simulink model "main_simulation_without_FKw"  (R2015a)
settings: Solver=ode45  StartTime=0.0  StopTime=10  FixedStep=1e-4  MaxStep=1e-3  RelTol=1e-3
values from neighbouring files (symbols this model uses):
  Ab11 = Ab(1:qw,1:qw)    [main_new.m]
  Ab12 = Ab(1:qw,qw+1:end)    [main_new.m]
  Ap = A    [main_new.m]
  Bb1 = Bb(1:qw,:)    [main_new.m]
  Bp = B    [main_new.m]
  Cb1p = (Cb1'*Cb1)^-1*Cb1'    [main_new.m]
  Cb2 = Cb(:,qw+1:end)    [main_new.m]
  Cp = C    [main_new.m]
  Ct = M*(eye(p)-Cb1*Cb1p)*Cb2    [main_new.m]
  Hp = H    [main_new.m]
  Ht = M*(eye(p)-Cb1*Cb1p)    [main_new.m]
  Kw = [0.158157916499 0.63846121775 -0.50742483629]    [Kw.mat]
  Kx = [0.978793467395 0.115253740456 -0.0372496439283 0.23631932633 2.68523757626 0.686096731216 0.555565644056 0.104452817235 0.744612452854 0.95412117755 0.434401201084 2.92090282506 ... (18 elements, 3x6)]    [Kx.mat]
  L = [732.974875612  -277.124666785; -145.685949536  40.2310279193; -21.3176025114  5.29309640103; -7.2125257354  1.1132328988; -36.4024893883  14.5426348186]    [L.mat]
  N = [-9.05549588116 -0.0761441556143 -0.0825387256676 0.135276633069 -0.0642378069483 -0.0761441556143 -9.64406895175 0.00880586634764 0.827985535249 0.695939837272 -0.0825387256676 0.00880586634764 ... (25 elements, 5x5)]    [N.mat]
  Q1 = Q(:,1:qw)    [main_new.m]
  Q2 = Q(:,qw+1:end)    [main_new.m]
  Sigma1 = Sigmaw(1:qw,:)    [main_new.m]
undefined symbols (not defined in the file or in its folder): C, J
libraries: dsparch4 x1
settings Model: Creator=p4wp4w  LastModifiedBy=p4wp4w

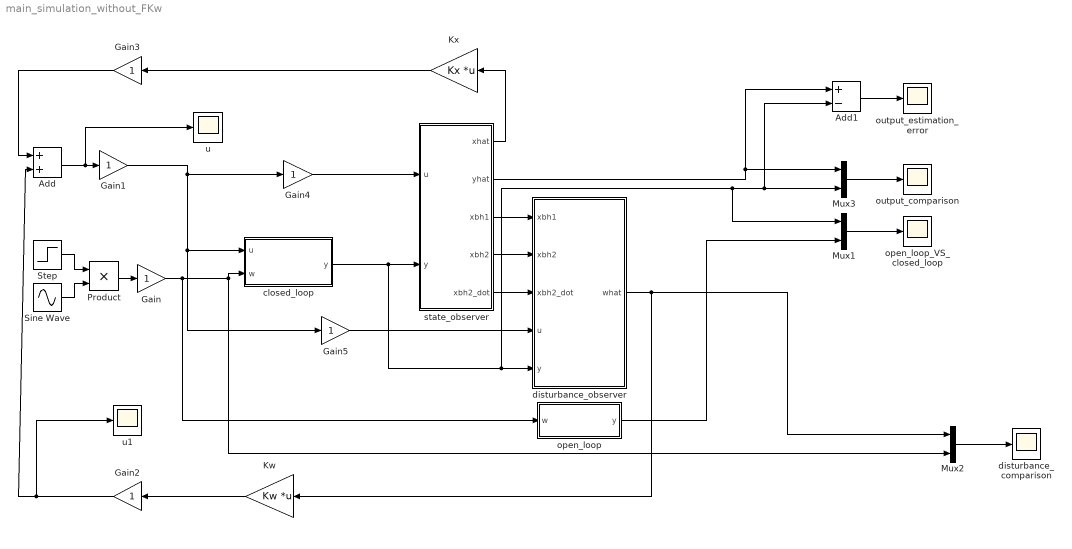
== system main_simulation_without_FKw ==
  Add : Sum
  Add1 : Sum  Inputs=+-
  Gain{,1..5} (6 alike) : Gain
  Kw : Gain  Gain=Kw  Multiplication=Matrix(K*u)
  Kx : Gain  Gain=Kx  Multiplication=Matrix(K*u)
  Mux1 : Mux  Inputs=2
  Mux2 : Mux  Inputs=2
  Mux3 : Mux  Inputs=2
  Product : Product
  Sine Wave : Sin  Frequency=10  SampleTime=0
  Step : Step  Time=5  Before=8  After=0  SampleTime=0
  closed_loop : Subsystem
  disturbance_comparison : Scope
      settings: YMin=-15  YMax=15
  disturbance_observer : Subsystem
  open_loop : Subsystem
  open_loop_VS_closed_loop : Scope
      settings: ShowLegends=on  YMin=-2.5e+09  YMax=3e+10  SaveName=ScopeData4
  output_comparison : Scope
      settings: YMin=-0.0024  YMax=-2.1684e-19
  output_estimation_error : Scope
      settings: YMin=-0.0024  YMax=-2.1684e-19  SaveName=ScopeData3
  state_observer : Subsystem
  u : Scope
      settings: SaveName=ScopeData2
  u1 : Scope
      settings: YMin=-2.5e+33  YMax=8.5e+33  SaveName=ScopeData5
  wires:
  Gain1/1 -> Gain5/1, closed_loop/1(u), Gain4/1
  closed_loop/1(y) -> Mux1/1, Add1/2, Mux3/2, disturbance_observer/5(y), state_observer/2(y)
  Mux2/1 -> disturbance_comparison/1
  state_observer/3(xbh1) -> disturbance_observer/1(xbh1)
  state_observer/4(xbh2) -> disturbance_observer/2(xbh2)
  state_observer/5(xbh2_dot) -> disturbance_observer/3(xbh2_dot)
  Mux3/1 -> output_comparison/1
  state_observer/2(yhat) -> Add1/1, Mux3/1
  disturbance_observer/1(what) -> Kw/1, Mux2/1
  Gain/1 -> open_loop/1(w), Mux2/2, closed_loop/2(w)
  state_observer/1(xhat) -> Kx/1
  Add/1 -> u/1, Gain1/1
  Kx/1 -> Gain3/1
  Kw/1 -> Gain2/1
  Gain2/1 -> u1/1, Add/2
  Gain3/1 -> Add/1
  Add1/1 -> output_estimation_error/1
  open_loop/1(y) -> Mux1/2
  Mux1/1 -> open_loop_VS_closed_loop/1
  Product/1 -> Gain/1
  Step/1 -> Product/1
  Sine Wave/1 -> Product/2
  Gain4/1 -> state_observer/1(u)
  Gain5/1 -> disturbance_observer/4(u)

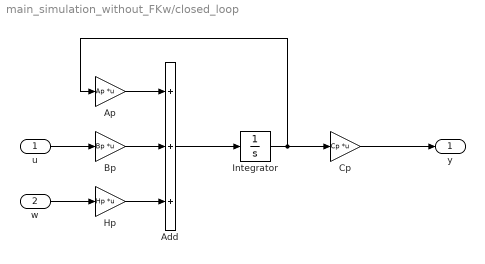
== system main_simulation_without_FKw/closed_loop ==
  u : Inport
  w : Inport  Port=2
  Add : Sum  Inputs=+++
  Ap : Gain  Gain=Ap  Multiplication=Matrix(K*u)
  Bp : Gain  Gain=Bp  Multiplication=Matrix(K*u)
  Cp : Gain  Gain=Cp  Multiplication=Matrix(K*u)
  Hp : Gain  Gain=Hp  Multiplication=Matrix(K*u)
  Integrator : Integrator
  y : Outport
  wires:
  w/1 -> Hp/1
  u/1 -> Bp/1
  Add/1 -> Integrator/1
  Bp/1 -> Add/2
  Integrator/1 -> Cp/1, Ap/1
  Ap/1 -> Add/1
  Hp/1 -> Add/3
  Cp/1 -> y/1

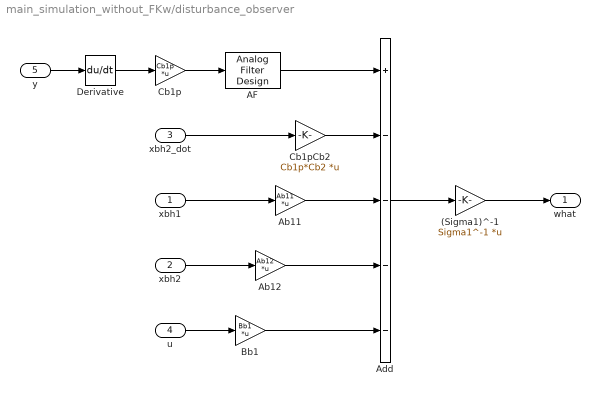
== system main_simulation_without_FKw/disturbance_observer ==
  xbh1 : Inport
  xbh2 : Inport  Port=2
  xbh2_dot : Inport  Port=3
  u : Inport  Port=4
  y : Inport  Port=5
  (Sigma1)^-1 : Gain  Gain=Sigma1^-1  Multiplication=Matrix(K*u)
  AF : dsparch4/Analog Filter Design  method=Butterworth  filttype=Lowpass  N=2  Wlo=30  Whi=80  Rp=2  Rs=40
  Ab11 : Gain  Gain=Ab11  Multiplication=Matrix(K*u)
  Ab12 : Gain  Gain=Ab12  Multiplication=Matrix(K*u)
  Add : Sum  Inputs=+----
  Bb1 : Gain  Gain=Bb1  Multiplication=Matrix(K*u)
  Cb1p : Gain  Gain=Cb1p  Multiplication=Matrix(K*u)
  Cb1pCb2 : Gain  Gain=Cb1p*Cb2  Multiplication=Matrix(K*u)
  Derivative : Derivative
  what : Outport
  wires:
  (Sigma1)^-1/1 -> what/1
  y/1 -> Derivative/1
  Derivative/1 -> Cb1p/1
  Add/1 -> (Sigma1)^-1/1
  Cb1pCb2/1 -> Add/2
  xbh2_dot/1 -> Cb1pCb2/1
  Ab11/1 -> Add/3
  xbh1/1 -> Ab11/1
  Ab12/1 -> Add/4
  xbh2/1 -> Ab12/1
  u/1 -> Bb1/1
  Bb1/1 -> Add/5
  Cb1p/1 -> AF/1
  AF/1 -> Add/1

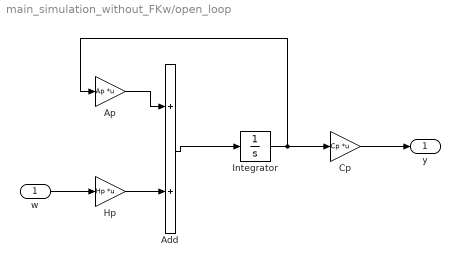
== system main_simulation_without_FKw/open_loop ==
  w : Inport
  Add : Sum
  Ap : Gain  Gain=Ap  Multiplication=Matrix(K*u)
  Cp : Gain  Gain=Cp  Multiplication=Matrix(K*u)
  Hp : Gain  Gain=Hp  Multiplication=Matrix(K*u)
  Integrator : Integrator
  y : Outport
  wires:
  Cp/1 -> y/1
  Hp/1 -> Add/2
  Ap/1 -> Add/1
  Integrator/1 -> Ap/1, Cp/1
  Add/1 -> Integrator/1
  w/1 -> Hp/1

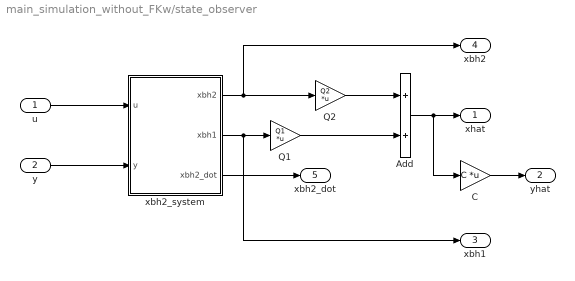
== system main_simulation_without_FKw/state_observer ==
  u : Inport
  y : Inport  Port=2
  Add : Sum
  C : Gain  Gain=C  Multiplication=Matrix(K*u)
  Q1 : Gain  Gain=Q1  Multiplication=Matrix(K*u)
  Q2 : Gain  Gain=Q2  Multiplication=Matrix(K*u)
  xbh2_system : Subsystem
  xhat : Outport
  yhat : Outport  Port=2
  xbh1 : Outport  Port=3
  xbh2 : Outport  Port=4
  xbh2_dot : Outport  Port=5
  wires:
  Add/1 -> C/1, xhat/1
  u/1 -> xbh2_system/1(u)
  y/1 -> xbh2_system/2(y)
  xbh2_system/1(xbh2) -> xbh2/1, Q2/1
  Q2/1 -> Add/1
  xbh2_system/2(xbh1) -> xbh1/1, Q1/1
  Q1/1 -> Add/2
  C/1 -> yhat/1
  xbh2_system/3(xbh2_dot) -> xbh2_dot/1

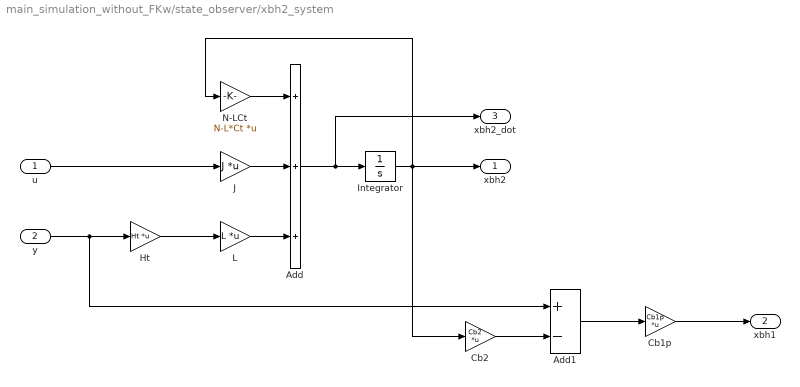
== system main_simulation_without_FKw/state_observer/xbh2_system ==
  u : Inport
  y : Inport  Port=2
  Add : Sum  Inputs=+++
  Add1 : Sum  Inputs=+-
  Cb1p : Gain  Gain=Cb1p  Multiplication=Matrix(K*u)
  Cb2 : Gain  Gain=Cb2  Multiplication=Matrix(K*u)
  Ht : Gain  Gain=Ht  Multiplication=Matrix(K*u)
  Integrator : Integrator
  J : Gain  Gain=J  Multiplication=Matrix(K*u)
  L : Gain  Gain=L  Multiplication=Matrix(K*u)
  N-LCt : Gain  Gain=N-L*Ct  Multiplication=Matrix(K*u)
  xbh2 : Outport
  xbh1 : Outport  Port=2
  xbh2_dot : Outport  Port=3
  wires:
  N-LCt/1 -> Add/1
  Integrator/1 -> Cb2/1, xbh2/1, N-LCt/1
  J/1 -> Add/2
  Add/1 -> xbh2_dot/1, Integrator/1
  u/1 -> J/1
  y/1 -> Add1/1, Ht/1
  L/1 -> Add/3
  Ht/1 -> L/1
  Add1/1 -> Cb1p/1
  Cb2/1 -> Add1/2
  Cb1p/1 -> xbh1/1
